simulink library "GearSystemsControl"  (R2023b)
settings: Solver=VariableStepAuto  StartTime=0.0  StopTime=10.0  RelTol=1e-3
undefined symbols (not defined in the file or in its folder): eta_EM_neg, eta_EM_pos, h, nr_gearsGL, P_opt_neg1, P_opt_neg2, P_opt_pos1, P_opt_pos2, T_EM_neg, T_EM_pos, w1, w1_n, w2S_n, w2S_p, w_EM_row
libraries: simulink x10
settings Model: Creator=dadikozyanaa  LastModifiedBy=ivank
settings DebuggingCC: UnconnectedInputMsg=warning  UnconnectedOutputMsg=warning  UnconnectedLineMsg=warning
settings ModelReferenceCC: EnableRefExpFcnMdlSchedulingChecks=on
settings RTWCC: DLArmComputeVersion=19.05

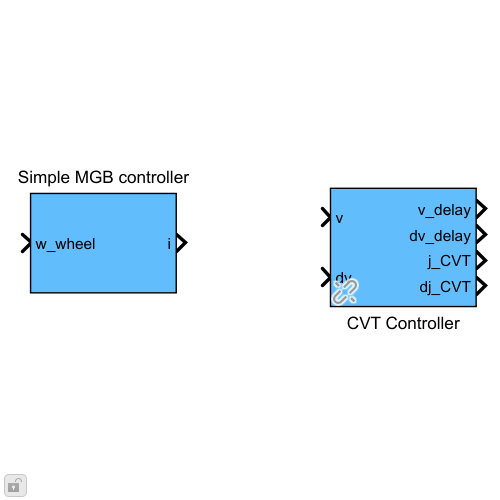
[thumbnail: Simulink's stored preview of the top-level diagram]
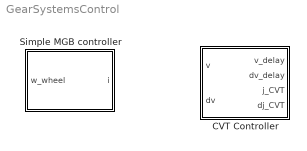
== system GearSystemsControl ==
  CVT Controller : Subsystem  Tag=cvt controller  AncestorBlock=GearSystemsControl/CVT Controller  mask(CVT Controller){j_CVT_min=3, j_CVT_max=15, w_wheel_min=3, w_CVT_idle=100, w_CVT_upper=300}
      mask prompts: j_CVT_min "Lower gear ratio limit [-]"; j_CVT_max "Upper gear ratio limit [-]"; w_wheel_min "Minimum wheel speed [rad/s]"; w_CVT_idle "CVT idle speed [rad/s]"; w_CVT_upper "Maximum CVT speed [rad/s]"
      mask help:
      | This block calculates the optimum gear ratio and its change during one integration step for a CVT.
      |
      | Input:
      | =====
      | 	v	Speed [m/s]
      | 	dv	Acceleration [m/s^2]
      |
      | Output:
      | ======
      | 	v_delay	Speed one step delayed [m/s]
      | 	dv_delay	Acceleration one step delayed [m/s^2]
      | 	j_CVT	Gear ratio [-]
      | 	dj_CVT	Change of gear ratio [1/s]
      mask init:
      | init_CVT_ctrl;
  Simple MGB controller : Subsystem  mask(Simple MGB controller){nr_gears=3, w_shift2=10, w_shift3=20, w_shift4=1e10, w_shift5=1e10, w_shift6=1e10}
      mask prompts: nr_gears "Select number of gears:"; w_shift2 "Threshold velocity gear 2 [rad/s]"; w_shift3 "Threshold velocity gear 3 [rad/s]"; w_shift4 "Threshold velocity gear 4 [rad/s]"; w_shift5 "Threshold velocity gear 5 [rad/s]"; w_shift6 "Threshold velocity gear 6 [rad/s]"
      mask help:
      | This block simulates a simple MGB controller.
      |
      | Input:
      | =====
      | 	w_wheel	Speed of the wheel [rad/s]
      |
      | Output:
      | ======
      | 	i	Gear number [-]
      mask init:
      | init_MGB_control;
      mask Help: Contact a.a.dadikozyan@student.tue.nl
      mask TypeOptions nr_gears: 2 | 3 | 4 | 5 | 6
      mask Callback nr_gears:
      | maskStr = get_param(gcb,'nr_gears');
      | 
      | switch maskStr
      |     case '2'
      |         set_param(gcb,'MaskVisibilities',{'on';'on';'off';'off';'off';'off'}),
      |         set_param(gcb,'w_shift3','1e10'),
      |         set_param(gcb,'w_shift4','1e10'),
      |         set_param(gcb,'w_shift5','1e10'),
      |         set_param(gcb,'w_shift6','1e10'),
      |     case '3'
      |         set_param(gcb,'MaskVisibilities',{'on';'on';'on';'off';'off';'off'}),
      |         set_param(gcb,'w_shift4','1e10'),
      |         set_param(gcb,'w_shift5','1e10'),
      |         set_param(gcb,'w_shift6','1e10'),
      |     case '4'
      |         set_param(gcb,'MaskVisibilities',{'on';'on';'on';'on';'off';'off'}),
      |         set_param(gcb,'w_shift5','1e10'),
      |         set_param(gcb,'w_shift6','1e10'),
      |     case '5'
      |         set_param(gcb,'MaskVisibilities',{'on';'on';'on';'on';'on';'off'}),
      |         set_param(gcb,'w_shift6','1e10'),
      |     case '6'
      |         set_param(gcb,'MaskVisibilities',{'on';'on';'on';'on';'on';'on'}),
      | end
      | 
      | %set_param(gcb,'editvalue',maskStr);

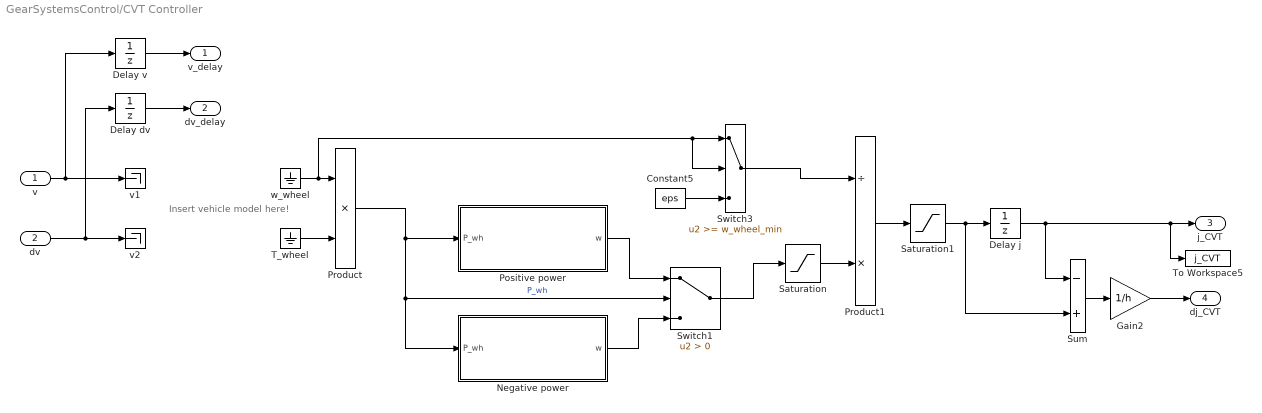
== system GearSystemsControl/CVT Controller ==
  note: Insert vehicle
      | model here!
  v : Inport
  dv : Inport  Port=2
  Constant5 : Constant  Value=eps
  Delay dv : UnitDelay  SampleTime=h
  Delay j : UnitDelay  InitialCondition=j_CVT_min  SampleTime=h
  Delay v : UnitDelay  SampleTime=h
  Gain2 : Gain  Gain=1/h  SaturateOnIntegerOverflow=on  OutDataTypeStr=Inherit: Same as input  ParamDataTypeStr=Inherit: Same as input
  Negative power : Subsystem
  Positive power : Subsystem
  Product : Product  InputSameDT=on  RndMeth=Zero  SaturateOnIntegerOverflow=on  OutDataTypeStr=Inherit: Same as first input
  Product1 : Product  Inputs=/*  InputSameDT=on  RndMeth=Zero  SaturateOnIntegerOverflow=on  OutDataTypeStr=Inherit: Same as first input
  Saturation : Saturate  UpperLimit=w_CVT_upper  LowerLimit=w_CVT_idle
  Saturation1 : Saturate  UpperLimit=j_CVT_max  LowerLimit=j_CVT_min
  Sum : Sum  Inputs=-+  InputSameDT=on  SaturateOnIntegerOverflow=on  OutDataTypeStr=Inherit: Same as first input
  Switch1 : Switch  Criteria=u2 > Threshold  SaturateOnIntegerOverflow=off  InputSameDT=off
  Switch3 : Switch  Threshold=w_wheel_min
  T_wheel : Ground
  To Workspace5 : ToWorkspace  VariableName=j_CVT  SampleTime=-1
  v1 : Terminator
  v2 : Terminator
  w_wheel : Ground
  v_delay : Outport  InitialOutput=0
  dv_delay : Outport  Port=2  InitialOutput=0
  j_CVT : Outport  Port=3  InitialOutput=0
  dj_CVT : Outport  Port=4  InitialOutput=0
  wires:
  Saturation/1 -> Product1/2
  Switch1/1 -> Saturation/1
  dv/1 -> Delay dv/1, v2/1
  Negative power/1(w) -> Switch1/3
  T_wheel/1 -> Product/2
  Delay v/1 -> v_delay/1
  Saturation1/1 -> Delay j/1, Sum/2
  Delay dv/1 -> dv_delay/1
  Delay j/1 -> To Workspace5/1, j_CVT/1, Sum/1
  Switch3/1 -> Product1/1
  Product/1 -> Positive power/1(P_wh), Negative power/1(P_wh), Switch1/2  "P_wh"
  Constant5/1 -> Switch3/3
  w_wheel/1 -> Product/1, Switch3/2, Switch3/1
  Sum/1 -> Gain2/1
  v/1 -> Delay v/1, v1/1
  Positive power/1(w) -> Switch1/1
  Product1/1 -> Saturation1/1
  Gain2/1 -> dj_CVT/1

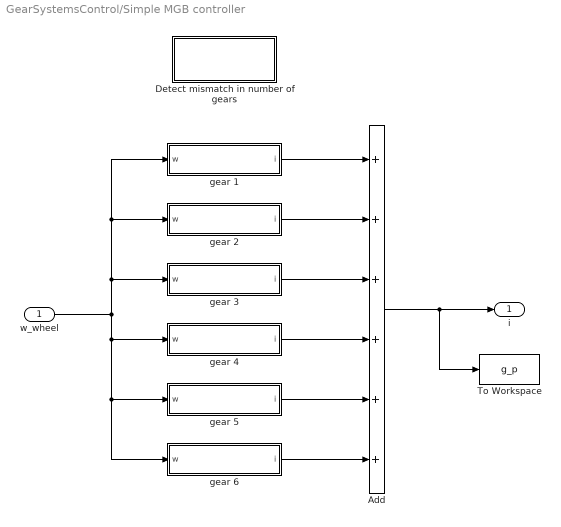
== system GearSystemsControl/Simple MGB controller ==
  w_wheel : Inport
  Add : Sum  Inputs=++++++
  Detect mismatch in number of gears : Subsystem
  To Workspace : ToWorkspace  VariableName=g_p  SampleTime=-1
  gear 1 : Subsystem
  gear 2 : Subsystem
  gear 3 : Subsystem
  gear 4 : Subsystem
  gear 5 : Subsystem
  gear 6 : Subsystem
  i : Outport
  wires:
  gear 6/1(i) -> Add/6
  Add/1 -> To Workspace/1, i/1
  gear 2/1(i) -> Add/2
  gear 4/1(i) -> Add/4
  gear 3/1(i) -> Add/3
  gear 5/1(i) -> Add/5
  gear 1/1(i) -> Add/1
  w_wheel/1 -> gear 4/1(w), gear 5/1(w), gear 6/1(w), gear 3/1(w), gear 2/1(w), gear 1/1(w)

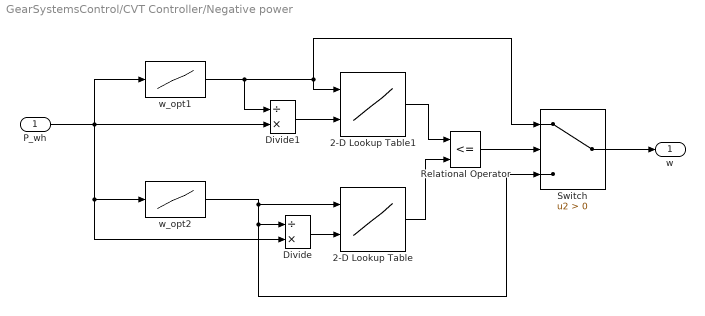
== system GearSystemsControl/CVT Controller/Negative power ==
  P_wh : Inport
  2-D Lookup Table : Lookup_n-D  BreakpointsForDimension1=T_EM_neg  BreakpointsForDimension2=w_EM_row  Table=eta_EM_neg  InternalRulePriority=Speed  RndMeth=Simplest
      settings: InputPortMap=u0,u1
  2-D Lookup Table1 : Lookup_n-D  BreakpointsForDimension1=T_EM_neg  BreakpointsForDimension2=w_EM_row  Table=eta_EM_neg  InternalRulePriority=Speed  RndMeth=Simplest
      settings: InputPortMap=u0,u1
  Divide : Product  Inputs=/*
  Divide1 : Product  Inputs=/*
  Relational Operator : RelationalOperator  Operator=<=  OutDataTypeStr=boolean  RndMeth=Simplest  InputSameDT=off
  Switch : Switch  Criteria=u2 > Threshold  SaturateOnIntegerOverflow=off  InputSameDT=off
  w_opt1 : Lookup  InputValues=P_opt_neg1  Table=w1_n
  w_opt2 : Lookup  InputValues=P_opt_neg2  Table=w2S_n
  w : Outport
  wires:
  Divide/1 -> 2-D Lookup Table/2
  2-D Lookup Table1/1 -> Relational Operator/1
  Switch/1 -> w/1
  w_opt1/1 -> Divide1/1, 2-D Lookup Table1/1, Switch/1
  P_wh/1 -> w_opt1/1, Divide1/2, w_opt2/1, Divide/2
  Divide1/1 -> 2-D Lookup Table1/2
  w_opt2/1 -> 2-D Lookup Table/1, Divide/1, Switch/3
  2-D Lookup Table/1 -> Relational Operator/2
  Relational Operator/1 -> Switch/2

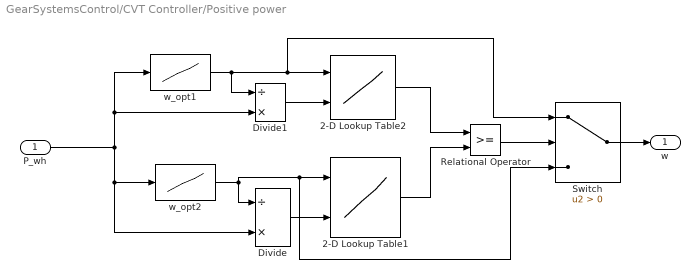
== system GearSystemsControl/CVT Controller/Positive power ==
  P_wh : Inport
  2-D Lookup Table1 : Lookup_n-D  BreakpointsForDimension1=T_EM_pos  BreakpointsForDimension2=w_EM_row  Table=eta_EM_pos  InternalRulePriority=Speed  RndMeth=Simplest
      settings: InputPortMap=u0,u1
  2-D Lookup Table2 : Lookup_n-D  BreakpointsForDimension1=T_EM_pos  BreakpointsForDimension2=w_EM_row  Table=eta_EM_pos  InternalRulePriority=Speed  RndMeth=Simplest
      settings: InputPortMap=u0,u1
  Divide : Product  Inputs=/*
  Divide1 : Product  Inputs=/*
  Relational Operator : RelationalOperator  OutDataTypeStr=boolean  RndMeth=Simplest  InputSameDT=off
  Switch : Switch  Criteria=u2 > Threshold  SaturateOnIntegerOverflow=off  InputSameDT=off
  w_opt1 : Lookup  InputValues=P_opt_pos1  Table=w1
  w_opt2 : Lookup  InputValues=P_opt_pos2  Table=w2S_p
  w : Outport
  wires:
  2-D Lookup Table2/1 -> Relational Operator/1
  Divide1/1 -> 2-D Lookup Table2/2
  2-D Lookup Table1/1 -> Relational Operator/2
  w_opt2/1 -> Switch/3, 2-D Lookup Table1/1, Divide/1
  Relational Operator/1 -> Switch/2
  Switch/1 -> w/1
  P_wh/1 -> w_opt1/1, Divide1/2, w_opt2/1, Divide/2
  w_opt1/1 -> Divide1/1, Switch/1, 2-D Lookup Table2/1
  Divide/1 -> 2-D Lookup Table1/2

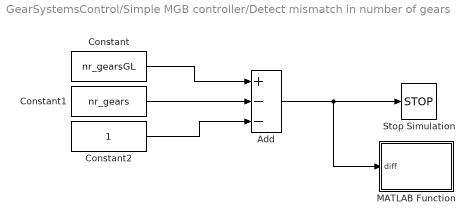
== system GearSystemsControl/Simple MGB controller/Detect mismatch in number of gears ==
  Add : Sum  Inputs=+--
  Constant : Constant  Value=nr_gearsGL
  Constant1 : Constant  Value=nr_gears
  Constant2 : Constant
  MATLAB Function : MATLAB Function  TreatAsAtomicUnit=on
  Stop Simulation : Stop
  wires:
  Constant/1 -> Add/1
  Constant1/1 -> Add/2
  Constant2/1 -> Add/3
  Add/1 -> MATLAB Function/1(diff), Stop Simulation/1

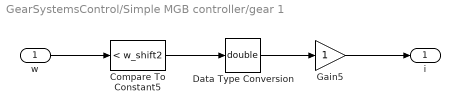
== system GearSystemsControl/Simple MGB controller/gear 1 ==
  w : Inport
  Compare To Constant5 : simulink/Logic and Bit Operations/Compare To Constant  relop=<  const=w_shift2  OutDataTypeStr=boolean
  Data Type Conversion : DataTypeConversion  OutDataTypeStr=double  SaturateOnIntegerOverflow=off  RndMeth=Floor
  Gain5 : Gain
  i : Outport
  wires:
  Data Type Conversion/1 -> Gain5/1
  Compare To Constant5/1 -> Data Type Conversion/1
  w/1 -> Compare To Constant5/1
  Gain5/1 -> i/1

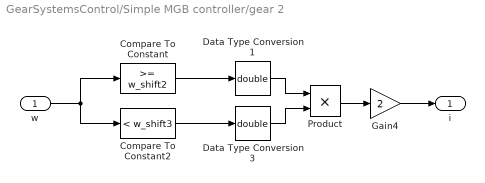
== system GearSystemsControl/Simple MGB controller/gear 2 ==
  w : Inport
  Compare To Constant : simulink/Logic and Bit Operations/Compare To Constant  relop=>=  const=w_shift2  OutDataTypeStr=boolean
  Compare To Constant2 : simulink/Logic and Bit Operations/Compare To Constant  relop=<  const=w_shift3  OutDataTypeStr=boolean
  Data Type Conversion1 : DataTypeConversion  OutDataTypeStr=double  SaturateOnIntegerOverflow=off  RndMeth=Floor
  Data Type Conversion3 : DataTypeConversion  OutDataTypeStr=double  SaturateOnIntegerOverflow=off  RndMeth=Floor
  Gain4 : Gain  Gain=2
  Product : Product
  i : Outport
  wires:
  Compare To Constant/1 -> Data Type Conversion1/1
  Compare To Constant2/1 -> Data Type Conversion3/1
  Data Type Conversion1/1 -> Product/1
  Product/1 -> Gain4/1
  Data Type Conversion3/1 -> Product/2
  Gain4/1 -> i/1
  w/1 -> Compare To Constant2/1, Compare To Constant/1

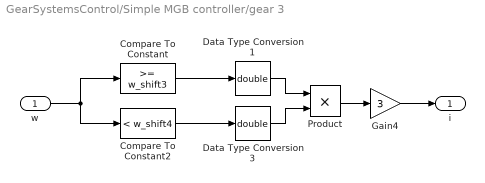
== system GearSystemsControl/Simple MGB controller/gear 3 ==
  w : Inport
  Compare To Constant : simulink/Logic and Bit Operations/Compare To Constant  relop=>=  const=w_shift3  OutDataTypeStr=boolean
  Compare To Constant2 : simulink/Logic and Bit Operations/Compare To Constant  relop=<  const=w_shift4  OutDataTypeStr=boolean
  Data Type Conversion1 : DataTypeConversion  OutDataTypeStr=double  SaturateOnIntegerOverflow=off  RndMeth=Floor
  Data Type Conversion3 : DataTypeConversion  OutDataTypeStr=double  SaturateOnIntegerOverflow=off  RndMeth=Floor
  Gain4 : Gain  Gain=3
  Product : Product
  i : Outport
  wires:
  Compare To Constant/1 -> Data Type Conversion1/1
  Compare To Constant2/1 -> Data Type Conversion3/1
  Data Type Conversion1/1 -> Product/1
  Product/1 -> Gain4/1
  Data Type Conversion3/1 -> Product/2
  Gain4/1 -> i/1
  w/1 -> Compare To Constant2/1, Compare To Constant/1

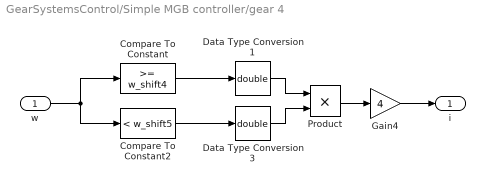
== system GearSystemsControl/Simple MGB controller/gear 4 ==
  w : Inport
  Compare To Constant : simulink/Logic and Bit Operations/Compare To Constant  relop=>=  const=w_shift4  OutDataTypeStr=boolean
  Compare To Constant2 : simulink/Logic and Bit Operations/Compare To Constant  relop=<  const=w_shift5  OutDataTypeStr=boolean
  Data Type Conversion1 : DataTypeConversion  OutDataTypeStr=double  SaturateOnIntegerOverflow=off  RndMeth=Floor
  Data Type Conversion3 : DataTypeConversion  OutDataTypeStr=double  SaturateOnIntegerOverflow=off  RndMeth=Floor
  Gain4 : Gain  Gain=4
  Product : Product
  i : Outport
  wires:
  Compare To Constant/1 -> Data Type Conversion1/1
  Compare To Constant2/1 -> Data Type Conversion3/1
  Data Type Conversion1/1 -> Product/1
  Product/1 -> Gain4/1
  Data Type Conversion3/1 -> Product/2
  Gain4/1 -> i/1
  w/1 -> Compare To Constant2/1, Compare To Constant/1

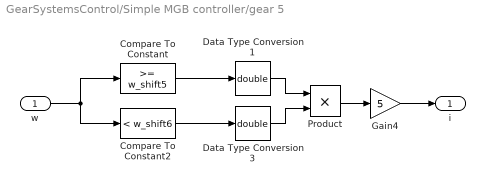
== system GearSystemsControl/Simple MGB controller/gear 5 ==
  w : Inport
  Compare To Constant : simulink/Logic and Bit Operations/Compare To Constant  relop=>=  const=w_shift5  OutDataTypeStr=boolean
  Compare To Constant2 : simulink/Logic and Bit Operations/Compare To Constant  relop=<  const=w_shift6  OutDataTypeStr=boolean
  Data Type Conversion1 : DataTypeConversion  OutDataTypeStr=double  SaturateOnIntegerOverflow=off  RndMeth=Floor
  Data Type Conversion3 : DataTypeConversion  OutDataTypeStr=double  SaturateOnIntegerOverflow=off  RndMeth=Floor
  Gain4 : Gain  Gain=5
  Product : Product
  i : Outport
  wires:
  Compare To Constant/1 -> Data Type Conversion1/1
  Compare To Constant2/1 -> Data Type Conversion3/1
  Data Type Conversion1/1 -> Product/1
  Product/1 -> Gain4/1
  Data Type Conversion3/1 -> Product/2
  Gain4/1 -> i/1
  w/1 -> Compare To Constant2/1, Compare To Constant/1

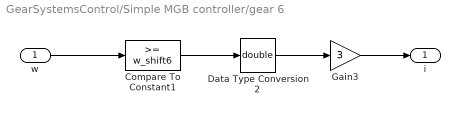
== system GearSystemsControl/Simple MGB controller/gear 6 ==
  w : Inport
  Compare To Constant1 : simulink/Logic and Bit Operations/Compare To Constant  relop=>=  const=w_shift6  OutDataTypeStr=boolean
  Data Type Conversion2 : DataTypeConversion  OutDataTypeStr=double  SaturateOnIntegerOverflow=off  RndMeth=Floor
  Gain3 : Gain  Gain=3
  i : Outport
  wires:
  Compare To Constant1/1 -> Data Type Conversion2/1
  Data Type Conversion2/1 -> Gain3/1
  Gain3/1 -> i/1
  w/1 -> Compare To Constant1/1

== matlab function GearSystemsControl/Simple MGB controller/Detect mismatch in number of gears/MATLAB Function ==
  data: diff input
function error_gears(diff)
if diff ~= 0
    error("Number of gears in transmission block and control block do not match!");
end
end
